simulink model "propagatorSimple"  (R2023b)
settings: Solver=VariableStepAuto  StartTime=0.0  StopTime=tf  RelTol=1e-8  AbsTol=1e-8
undefined symbols (not defined in the file or in its folder): area, burnOverride, initMass, juliandate, ref, thrust, thrustingThreshold
libraries: vrlib x4, simulink x1
settings Model: SimulationMode=rapid-accelerator  Creator=miqui  LastModifiedBy=miqui

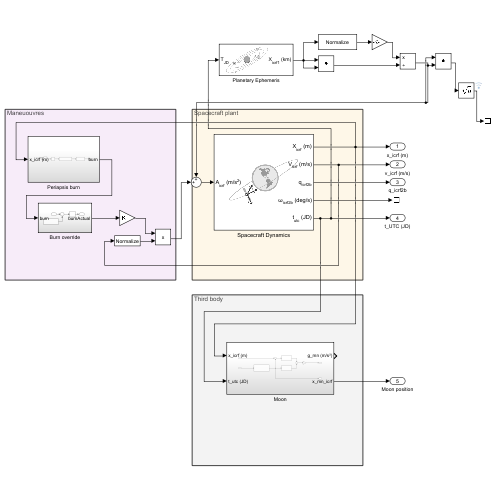
[thumbnail: Simulink's stored preview of the top-level diagram]
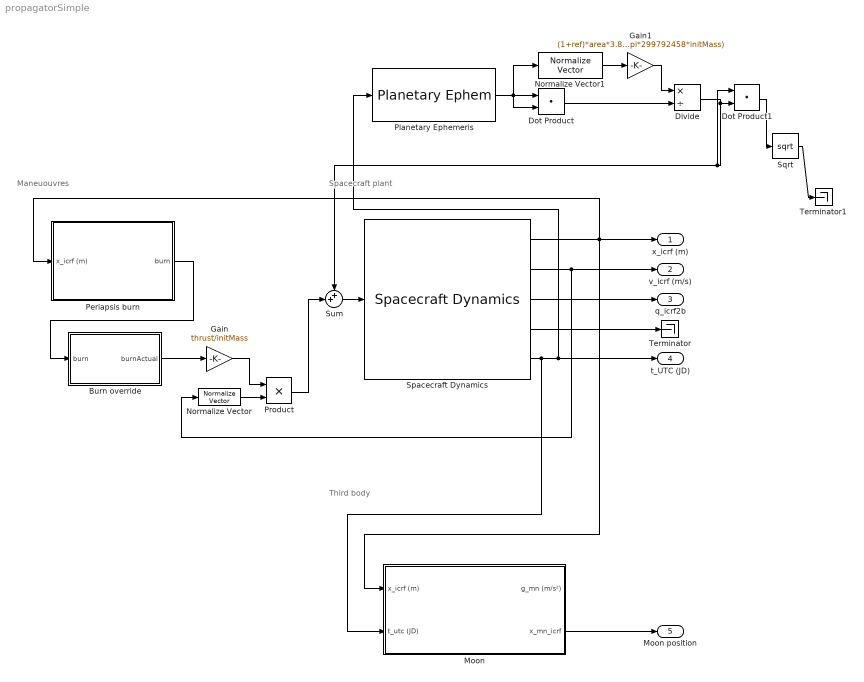
== system propagatorSimple ==
  note: Spacecraft plant
  note: Third body
  note: Maneuouvres
  Burn override : Subsystem
  Divide : Product  Inputs=*/
  Dot Product : DotProduct  OutDataTypeStr=Inherit: Inherit via internal rule
  Dot Product1 : DotProduct  OutDataTypeStr=Inherit: Inherit via internal rule
  Gain : Gain  Gain=thrust/initMass
  Gain1 : Gain  Gain=(1+ref)*area*3.852e26/(4*pi*299792458*initMass)
  Moon : Subsystem
  Normalize Vector : vrlib/Utilities/Normalize Vector  maxzero=0
  Normalize Vector1 : vrlib/Utilities/Normalize Vector  maxzero=0
  Periapsis burn : Subsystem
  Planetary Ephemeris : PlanetaryEphem  center=Sun  target=Earth  outputVelocity=off
  Product : Product
  Spacecraft Dynamics : SpacecraftDynamics  forcesIn=off  momentsIn=off  accelIn=on  startDate=startDate  mass=initMass  inertia=[1, 0, 0; 0, 1, 0; 0, 0, 1]*initMass  useMassFlowRelativeVelocity=on  semiMajorAxis=sma  eccentricity=ecc  inclination=inc  raan=RAAN  argPeriapsis=aop  trueAnomaly=true_an  gravityModel=Point-mass  useEOPs=off  useThirdBodyGravity=on  reflectivityCoeff=ref  srpArea=area
  Sqrt : Sqrt
  Sum : Sum  Inputs=++|
  Terminator : Terminator
  Terminator1 : Terminator
  x_icrf (m) : Outport
  v_icrf (m/s) : Outport  Port=2
  q_icrf2b : Outport  Port=3
  t_UTC (JD) : Outport  Port=4
  Moon position : Outport  Port=5
  wires:
  Spacecraft Dynamics/3 -> q_icrf2b/1
  Spacecraft Dynamics/2 -> Normalize Vector/1, v_icrf (m/s)/1
  Spacecraft Dynamics/5 -> Planetary Ephemeris/1, t_UTC (JD)/1, Moon/2(t_utc (JD))
  Moon/2(x_mn_icrf) -> Moon position/1
  Spacecraft Dynamics/4 -> Terminator/1
  Spacecraft Dynamics/1 -> Periapsis burn/1(x_icrf (m)), Moon/1(x_icrf (m)), x_icrf (m)/1
  Gain/1 -> Product/1
  Normalize Vector/1 -> Product/2
  Burn override/1(burnActual) -> Gain/1
  Periapsis burn/1(burn) -> Burn override/1(burn)
  Planetary Ephemeris/1 -> Normalize Vector1/1, Dot Product/2, Dot Product/1
  Normalize Vector1/1 -> Gain1/1
  Dot Product/1 -> Divide/2
  Gain1/1 -> Divide/1
  Sum/1 -> Spacecraft Dynamics/1
  Product/1 -> Sum/2
  Divide/1 -> Sum/1, Dot Product1/1, Dot Product1/2
  Dot Product1/1 -> Sqrt/1
  Sqrt/1 -> Terminator1/1

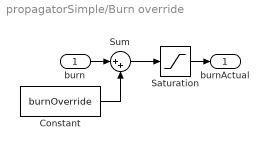
== system propagatorSimple/Burn override ==
  burn : Inport
  Constant : Constant  Value=burnOverride
  Saturation : Saturate  UpperLimit=1  LowerLimit=0
  Sum : Sum  Inputs=|++
  burnActual : Outport
  wires:
  Constant/1 -> Sum/2
  Saturation/1 -> burnActual/1
  burn/1 -> Sum/1
  Sum/1 -> Saturation/1

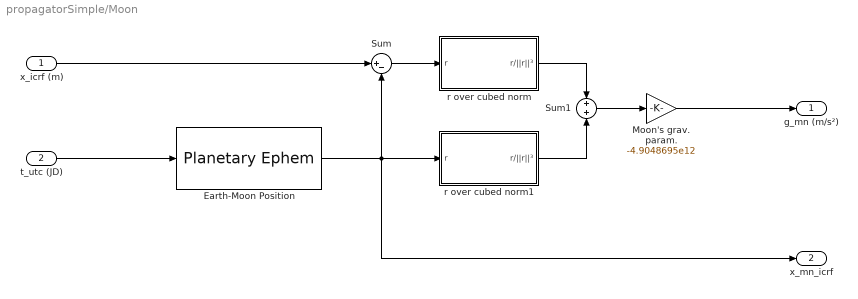
== system propagatorSimple/Moon ==
  x_icrf (m) : Inport
  t_utc (JD) : Inport  Port=2
  Earth-Moon Position : PlanetaryEphem  units=m,m/s  useDateRange=on  startDate=juliandate(2020,1,1)  outputVelocity=off
  Moon's grav. param. : Gain  Gain=-4.9048695e12
  Sum : Sum  Inputs=|+-
  Sum1 : Sum
  r over cubed norm : Subsystem
  r over cubed norm1 : Subsystem
  g_mn (m/s²) : Outport
  x_mn_icrf : Outport  Port=2
  wires:
  x_icrf (m)/1 -> Sum/1
  Earth-Moon Position/1 -> x_mn_icrf/1, r over cubed norm1/1(r), Sum/2
  Sum/1 -> r over cubed norm/1(r)
  Sum1/1 -> Moon's grav. param./1
  Moon's grav. param./1 -> g_mn (m/s²)/1
  r over cubed norm/1(r/||r||³) -> Sum1/1
  r over cubed norm1/1(r/||r||³) -> Sum1/2
  t_utc (JD)/1 -> Earth-Moon Position/1

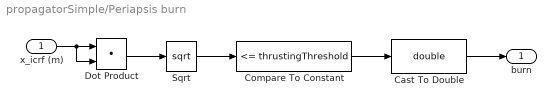
== system propagatorSimple/Periapsis burn ==
  x_icrf (m) : Inport
  Cast To Double : DataTypeConversion  OutDataTypeStr=double  SaturateOnIntegerOverflow=off  RndMeth=Floor
  Compare To Constant : simulink/Logic and Bit Operations/Compare To Constant  relop=<=  const=thrustingThreshold  OutDataTypeStr=boolean
  Dot Product : DotProduct  OutDataTypeStr=Inherit: Inherit via internal rule
  Sqrt : Sqrt
  burn : Outport
  wires:
  Dot Product/1 -> Sqrt/1
  Sqrt/1 -> Compare To Constant/1
  x_icrf (m)/1 -> Dot Product/2, Dot Product/1
  Compare To Constant/1 -> Cast To Double/1
  Cast To Double/1 -> burn/1

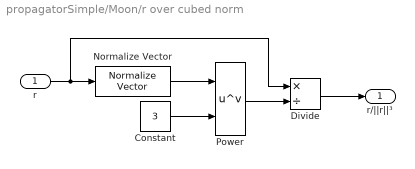
== system propagatorSimple/Moon/r over cubed norm ==
  r : Inport
  Constant : Constant  Value=3
  Divide : Product  Inputs=*/
  Normalize Vector : vrlib/Utilities/Normalize Vector  maxzero=0
  Power : Math  Operator=pow
  r/||r||³ : Outport
  wires:
  r/1 -> Divide/1, Normalize Vector/1
  Normalize Vector/1 -> Power/1
  Constant/1 -> Power/2
  Power/1 -> Divide/2
  Divide/1 -> r/||r||³/1

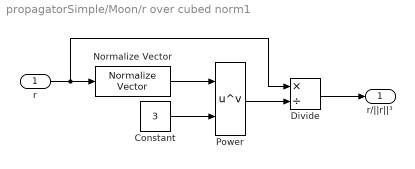
== system propagatorSimple/Moon/r over cubed norm1 ==
  r : Inport
  Constant : Constant  Value=3
  Divide : Product  Inputs=*/
  Normalize Vector : vrlib/Utilities/Normalize Vector  maxzero=0
  Power : Math  Operator=pow
  r/||r||³ : Outport
  wires:
  r/1 -> Divide/1, Normalize Vector/1
  Normalize Vector/1 -> Power/1
  Constant/1 -> Power/2
  Power/1 -> Divide/2
  Divide/1 -> r/||r||³/1
